simulink model "Guidance_ASMC_T1"  (R2020a)
settings: Solver=ode1  StartTime=0.0  StopTime=120  FixedStep=0.001  RelTol=1e-3
values from neighbouring files (symbols this model uses):
  trayectoria1 = [0 7 15 22 27 30 35 50 57 64 71 78 ... (76 elements, 19x4)]    [Points_T1.mat]
libraries: simulink x5
settings Model: Creator=franc  LastModifiedBy=Sebas
settings SolverCC: ZeroCrossAlgorithm=Adaptive
settings DebuggingCC: IgnoredZcDiagnostic=none
settings ModelReferenceCC: ModelReferenceMinAlgLoopOccurrences=on

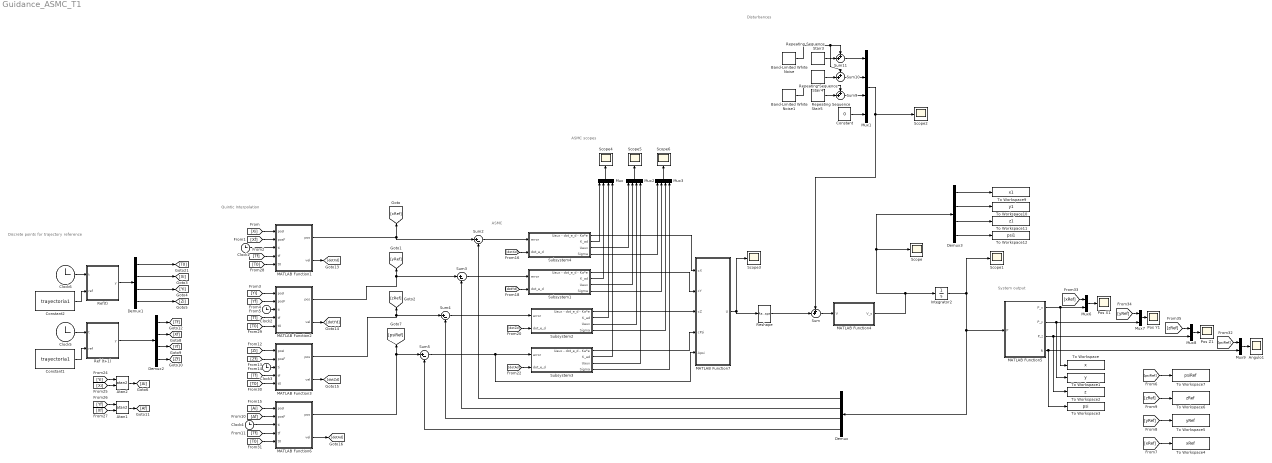
== system Guidance_ASMC_T1 ==
  note: ASMC scopes
  note: Quintic Interpolation
  note: Discrete points for trajectory reference
  note: System output
  note: ASMC
  note: Disturbances
  Angulo1 : Scope
  Atan1 : Trigonometry  Operator=atan2
  Atan2 : Trigonometry  Operator=atan2
  Band-Limited White Noise : simulink/Sources/Band-Limited White Noise  Cov=[1]  Ts=3  seed=[23341]
  Band-Limited White Noise1 : simulink/Sources/Band-Limited White Noise  Cov=[0.5]  Ts=12  seed=[23341]
  Clock{1..6} (6 alike) : Clock
  Constant : Constant  Value=0
  Constant1 : Constant  Value=trayectoria1
  Constant2 : Constant  Value=trayectoria1
  Demux{,1..3} (4 alike) : Demux
  Integrator2 : Integrator
  MATLAB Function1 : MATLAB Function  TreatAsAtomicUnit=on
  MATLAB Function2 : MATLAB Function  TreatAsAtomicUnit=on
  MATLAB Function3 : MATLAB Function  TreatAsAtomicUnit=on
  MATLAB Function4 : MATLAB Function  TreatAsAtomicUnit=on
      settings: MinAlgLoopOccurrences=on
  MATLAB Function5 : MATLAB Function  TreatAsAtomicUnit=on
  MATLAB Function6 : MATLAB Function  TreatAsAtomicUnit=on
  MATLAB Function7 : MATLAB Function  TreatAsAtomicUnit=on
      settings: MinAlgLoopOccurrences=on
  Mux{,1..3} (4 alike) : Mux
  Mux{6..9} (4 alike) : Mux  Inputs=2
  Pos X1 : Scope
  Pos Y1 : Scope
  Pos Z1 : Scope
  Ref (t+1) : MATLAB Function  TreatAsAtomicUnit=on  SystemSampleTime=1
  Ref(t) : MATLAB Function  TreatAsAtomicUnit=on  SystemSampleTime=1
  Repeating Sequence Stair3 : simulink/Sources/Repeating Sequence Stair  OutValues=[1 0.5 -1 -2 -0.5].'  tsamp=24  OutMin=[]  OutMax=[]  OutDataTypeStr=double  OutputDataTypeScalingMode=double  OutDataType=fixdt(0,8)  ConRadixGroup=Best Precision: Vector-wise  OutScaling=2^-12
  Repeating Sequence Stair4 : simulink/Sources/Repeating Sequence Stair  OutValues=[-1 -2 -1.5 -0.5 1].'  tsamp=24  OutMin=[]  OutMax=[]  OutDataTypeStr=double  OutputDataTypeScalingMode=double  OutDataType=fixdt(0,8)  ConRadixGroup=Best Precision: Vector-wise  OutScaling=2^-12
  Repeating Sequence Stair5 : simulink/Sources/Repeating Sequence Stair  OutValues=[0 -0.2 -0.4 -0.6 0].'  tsamp=24  OutMin=[]  OutMax=[]  OutDataTypeStr=double  OutputDataTypeScalingMode=double  OutDataType=fixdt(0,8)  ConRadixGroup=Best Precision: Vector-wise  OutScaling=2^-12
  Reshape : Reshape  OutputDimensionality=Customize  OutputDimensions=[4,1]
  Scope{,1..6} (7 alike) : Scope
  Subsystem1 : Subsystem  mask{Ka=1, K2=1, Beta=1, Mu=0.01}
  Subsystem2 : Subsystem  mask{Ka=2, K2=1, Beta=1, Mu=0.01}
  Subsystem3 : Subsystem  mask{Ka=1, K2=1, Beta=1, Mu=0.01}
  Subsystem4 : Subsystem  mask{Ka=1, K2=1, Beta=1, Mu=0.01}
  Sum{,9..11} (4 alike) : Sum  Inputs=++|
  Sum{2..5} (4 alike) : Sum  Inputs=|+-
  To Workspace : ToWorkspace  VariableName=x  SampleTime=-1
      settings: Save2DSignal=2-D array (concatenate along first dimension)
  To Workspace1 : ToWorkspace  VariableName=y  SampleTime=-1
      settings: Save2DSignal=2-D array (concatenate along first dimension)
  To Workspace10 : ToWorkspace  VariableName=y1  SampleTime=-1
      settings: Save2DSignal=2-D array (concatenate along first dimension)
  To Workspace11 : ToWorkspace  VariableName=z1  SampleTime=-1
      settings: Save2DSignal=2-D array (concatenate along first dimension)
  To Workspace12 : ToWorkspace  VariableName=psi1  SampleTime=-1
      settings: Save2DSignal=2-D array (concatenate along first dimension)
  To Workspace2 : ToWorkspace  VariableName=z  SampleTime=-1
      settings: Save2DSignal=2-D array (concatenate along first dimension)
  To Workspace3 : ToWorkspace  VariableName=psi  SampleTime=-1
      settings: Save2DSignal=2-D array (concatenate along first dimension)
  To Workspace4 : ToWorkspace  VariableName=xRef  SampleTime=-1
      settings: Save2DSignal=2-D array (concatenate along first dimension)
  To Workspace5 : ToWorkspace  VariableName=yRef  SampleTime=-1
      settings: Save2DSignal=2-D array (concatenate along first dimension)
  To Workspace6 : ToWorkspace  VariableName=zRef  SampleTime=-1
      settings: Save2DSignal=2-D array (concatenate along first dimension)
  To Workspace7 : ToWorkspace  VariableName=psiRef  SampleTime=-1
      settings: Save2DSignal=2-D array (concatenate along first dimension)
  To Workspace9 : ToWorkspace  VariableName=x1  SampleTime=-1
      settings: Save2DSignal=2-D array (concatenate along first dimension)
  wires:
  MATLAB Function5/1(P_x) -> Mux6/2, To Workspace/1
  MATLAB Function5/2(P_y) -> Mux7/2, To Workspace1/1
  MATLAB Function5/3(P_z) -> To Workspace2/1, Mux8/2
  MATLAB Function5/4(R) -> Mux9/2, To Workspace3/1
  Mux6/1 -> Pos X1/1
  Mux7/1 -> Pos Y1/1
  Mux8/1 -> Pos Z1/1
  Mux9/1 -> Angulo1/1
  MATLAB Function1/1(pos) -> [xRef], Sum2/1
  MATLAB Function3/1(pos) -> Sum4/1, [zRef]
  MATLAB Function6/1(pos) -> [psiRef], Sum5/1
  MATLAB Function2/1(pos) -> Sum3/1, [yRef]
  [xRef] -> To Workspace4/1
  [yRef] -> To Workspace5/1
  [psiRef] -> To Workspace7/1
  [zRef] -> To Workspace6/1
  [Tf] -> MATLAB Function6/4(tf)
  Clock4/1 -> MATLAB Function6/3(ti)
  [Ai] -> MATLAB Function6/1(posI)
  Demux1/3 -> [Yi]
  [Yf] -> MATLAB Function2/2(posF)
  Clock2/1 -> MATLAB Function2/3(ti)
  [Xi] -> MATLAB Function1/1(posI)
  [Af] -> MATLAB Function6/2(posF)
  [Yi] -> MATLAB Function2/1(posI)
  Demux1/2 -> [Xi]
  Demux2/1 -> [Tf]
  [Tf] -> MATLAB Function2/4(tf)
  Demux1/1 -> [T0]
  [Tf] -> MATLAB Function1/4(tf)
  Demux2/4 -> [Zf]
  Clock1/1 -> MATLAB Function1/3(ti)
  [Tf] -> MATLAB Function3/4(tf)
  [Zf] -> MATLAB Function3/2(posF)
  Clock3/1 -> MATLAB Function3/3(ti)
  [Xf] -> MATLAB Function1/2(posF)
  Demux2/3 -> [Yf]
  [Zi] -> MATLAB Function3/1(posI)
  Demux2/2 -> [Xf]
  MATLAB Function1/2(vel) -> [dotXd]
  MATLAB Function2/2(vel) -> [dotYd]
  MATLAB Function3/2(vel) -> [dotZd]
  MATLAB Function6/2(vel) -> [dotAd]
  Clock5/1 -> Ref (t+1)/1(t)
  Constant1/1 -> Ref (t+1)/2(ref)
  Constant2/1 -> Ref(t)/2(ref)
  Clock6/1 -> Ref(t)/1(t)
  Atan2/1 -> [Ai]
  [Xi] -> Atan2/2
  [Yi] -> Atan2/1
  Atan1/1 -> [Af]
  [Xf] -> Atan1/2
  [Yf] -> Atan1/1
  Ref (t+1)/1(y) -> Demux2/1
  Ref(t)/1(y) -> Demux1/1
  Demux1/4 -> [Zi]
  [T0] -> MATLAB Function1/5(t0)
  [T0] -> MATLAB Function2/5(t0)
  [T0] -> MATLAB Function3/5(t0)
  [T0] -> MATLAB Function6/5(t0)
  [xRef] -> Mux6/1
  [yRef] -> Mux7/1
  [zRef] -> Mux8/1
  [psiRef] -> Mux9/1
  Integrator2/1 -> Scope1/1, Demux/1, MATLAB Function5/1(P)
  Demux/1 -> Sum2/2
  Demux/2 -> Sum3/2
  MATLAB Function7/1(U) -> Reshape/1, Scope3/1
  [dotXd] -> Subsystem4/2(dot_e_d)
  Sum2/1 -> Subsystem4/1(error)
  Sum3/1 -> Subsystem1/1(error)
  Sum4/1 -> Subsystem2/1(error)
  [dotYd] -> Subsystem1/2(dot_e_d)
  [dotZd] -> Subsystem2/2(dot_e_d)
  [dotAd] -> Subsystem3/2(dot_e_d)
  Subsystem4/1(Uaux - dot_e_d - Ka*e) -> MATLAB Function7/1(cX)
  Subsystem1/1(Uaux - dot_e_d - Ka*e) -> MATLAB Function7/2(cY)
  Subsystem2/1(Uaux - dot_e_d - Ka*e) -> MATLAB Function7/3(cZ)
  Subsystem3/1(Uaux - dot_e_d - Ka*e) -> MATLAB Function7/4(cPsi)
  Demux/3 -> Sum4/2
  Demux/4 -> Sum5/2
  Sum5/1 -> Subsystem3/1(error), MATLAB Function7/5(Apsi)
  Sum/1 -> MATLAB Function4/1(V)
  Reshape/1 -> Sum/2
  Sum11/1 -> Mux1/1
  Repeating Sequence Stair4/1 -> Sum10/2
  Sum9/1 -> Mux1/3
  Sum10/1 -> Mux1/2
  Repeating Sequence Stair3/1 -> Sum11/2
  Mux1/1 -> Sum/1, Scope2/1
  Repeating Sequence Stair5/1 -> Sum9/2
  Constant/1 -> Mux1/4
  Band-Limited White Noise/1 -> Sum11/1, Sum10/1
  Band-Limited White Noise1/1 -> Sum9/1
  Demux3/2 -> To Workspace10/1
  Demux3/3 -> To Workspace11/1
  Demux3/4 -> To Workspace12/1
  MATLAB Function4/1(V_s) -> Scope/1, Demux3/1, Integrator2/1
  Demux3/1 -> To Workspace9/1
  Subsystem4/2(K_ad) -> Mux/1
  Subsystem1/2(K_ad) -> Mux/2
  Subsystem2/2(K_ad) -> Mux/3
  Subsystem3/2(K_ad) -> Mux/4
  Subsystem4/3(Uaux) -> Mux2/1
  Subsystem1/3(Uaux) -> Mux2/2
  Subsystem2/3(Uaux) -> Mux2/3
  Subsystem3/3(Uaux) -> Mux2/4
  Subsystem4/4(Sigma) -> Mux3/1
  Subsystem1/4(Sigma) -> Mux3/2
  Subsystem2/4(Sigma) -> Mux3/3
  Subsystem3/4(Sigma) -> Mux3/4
  Mux/1 -> Scope4/1
  Mux2/1 -> Scope5/1
  Mux3/1 -> Scope6/1

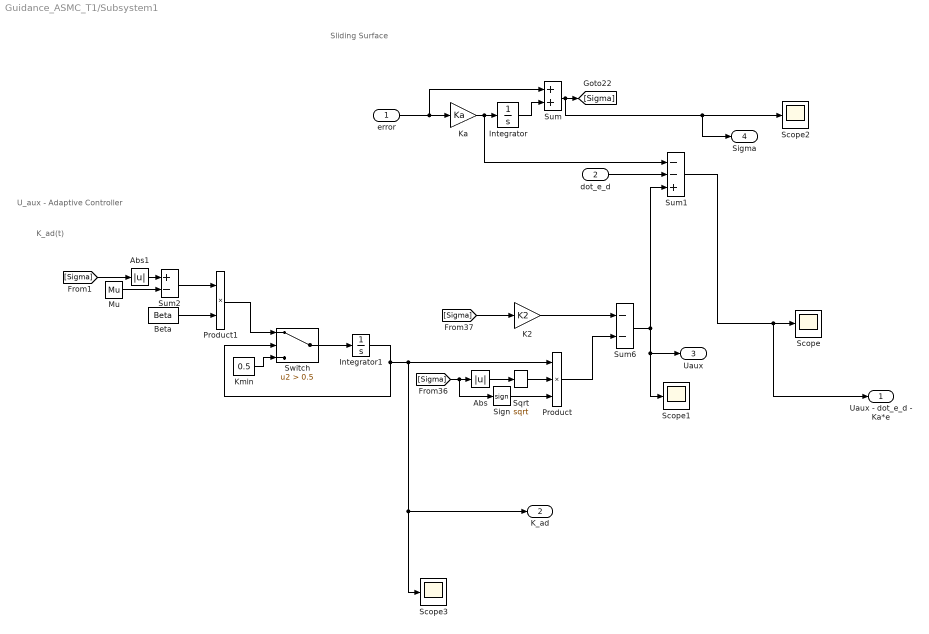
== system Guidance_ASMC_T1/Subsystem1 ==
  note: U_aux - Adaptive Controller
  note: Sliding Surface
  note: K_ad(t)
  error : Inport
  dot_e_d : Inport  Port=2
  Abs : Abs
  Abs1 : Abs
  Beta : Constant  Value=Beta
  Integrator : Integrator
  Integrator1 : Integrator
  K2 : Gain  Gain=K2
  Ka : Gain  Gain=Ka
  Kmin : Constant  Value=0.5
  Mu : Constant  Value=Mu
  Product : Product  Inputs=3
  Product1 : Product
  Scope{,1..3} (4 alike) : Scope
  Sign : Signum
  Sqrt : Sqrt  SaturateOnIntegerOverflow=on
  Sum : Sum
  Sum1 : Sum  Inputs=--+
  Sum2 : Sum  Inputs=+-
  Sum6 : Sum  Inputs=--
  Switch : Switch  Criteria=u2 > Threshold  Threshold=0.5
  Uaux - dot_e_d - Ka*e : Outport
  K_ad : Outport  Port=2
  Uaux : Outport  Port=3
  Sigma : Outport  Port=4
  wires:
  Integrator/1 -> Sum/2
  error/1 -> Sum/1, Ka/1
  [Sigma] -> K2/1
  Ka/1 -> Sum1/1, Integrator/1
  Sum6/1 -> Scope1/1, Uaux/1, Sum1/3
  [Sigma] -> Sign/1, Abs/1
  Product/1 -> Sum6/2
  Abs/1 -> Sqrt/1
  K2/1 -> Sum6/1
  Sum/1 -> Sigma/1, Scope2/1, [Sigma]
  Sign/1 -> Product/3
  Sqrt/1 -> Product/2
  Sum1/1 -> Uaux - dot_e_d - Ka*e/1, Scope/1
  dot_e_d/1 -> Sum1/2
  Switch/1 -> Integrator1/1
  Integrator1/1 -> Scope3/1, K_ad/1, Product/1, Switch/2
  Kmin/1 -> Switch/3
  [Sigma] -> Abs1/1
  Abs1/1 -> Sum2/1
  Mu/1 -> Sum2/2
  Beta/1 -> Product1/2
  Sum2/1 -> Product1/1
  Product1/1 -> Switch/1

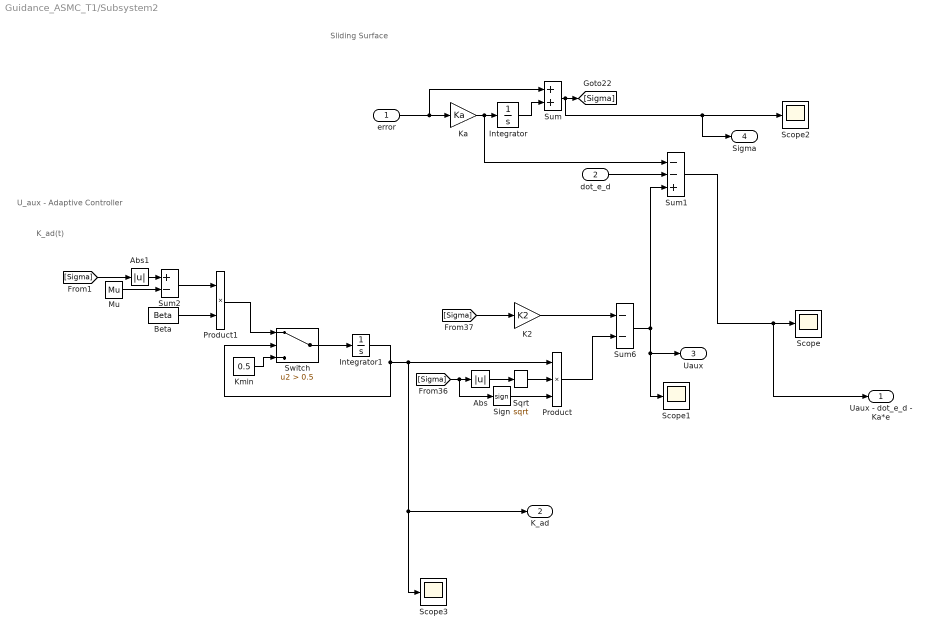
== system Guidance_ASMC_T1/Subsystem2 ==
  note: U_aux - Adaptive Controller
  note: Sliding Surface
  note: K_ad(t)
  error : Inport
  dot_e_d : Inport  Port=2
  Abs : Abs
  Abs1 : Abs
  Beta : Constant  Value=Beta
  Integrator : Integrator
  Integrator1 : Integrator
  K2 : Gain  Gain=K2
  Ka : Gain  Gain=Ka
  Kmin : Constant  Value=0.5
  Mu : Constant  Value=Mu
  Product : Product  Inputs=3
  Product1 : Product
  Scope{,1..3} (4 alike) : Scope
  Sign : Signum
  Sqrt : Sqrt  SaturateOnIntegerOverflow=on
  Sum : Sum
  Sum1 : Sum  Inputs=--+
  Sum2 : Sum  Inputs=+-
  Sum6 : Sum  Inputs=--
  Switch : Switch  Criteria=u2 > Threshold  Threshold=0.5
  Uaux - dot_e_d - Ka*e : Outport
  K_ad : Outport  Port=2
  Uaux : Outport  Port=3
  Sigma : Outport  Port=4
  wires:
  Integrator/1 -> Sum/2
  error/1 -> Sum/1, Ka/1
  [Sigma] -> K2/1
  Ka/1 -> Sum1/1, Integrator/1
  Sum6/1 -> Scope1/1, Uaux/1, Sum1/3
  [Sigma] -> Sign/1, Abs/1
  Product/1 -> Sum6/2
  Abs/1 -> Sqrt/1
  K2/1 -> Sum6/1
  Sum/1 -> Sigma/1, Scope2/1, [Sigma]
  Sign/1 -> Product/3
  Sqrt/1 -> Product/2
  Sum1/1 -> Uaux - dot_e_d - Ka*e/1, Scope/1
  dot_e_d/1 -> Sum1/2
  Switch/1 -> Integrator1/1
  Integrator1/1 -> Scope3/1, K_ad/1, Product/1, Switch/2
  Kmin/1 -> Switch/3
  [Sigma] -> Abs1/1
  Abs1/1 -> Sum2/1
  Mu/1 -> Sum2/2
  Beta/1 -> Product1/2
  Sum2/1 -> Product1/1
  Product1/1 -> Switch/1

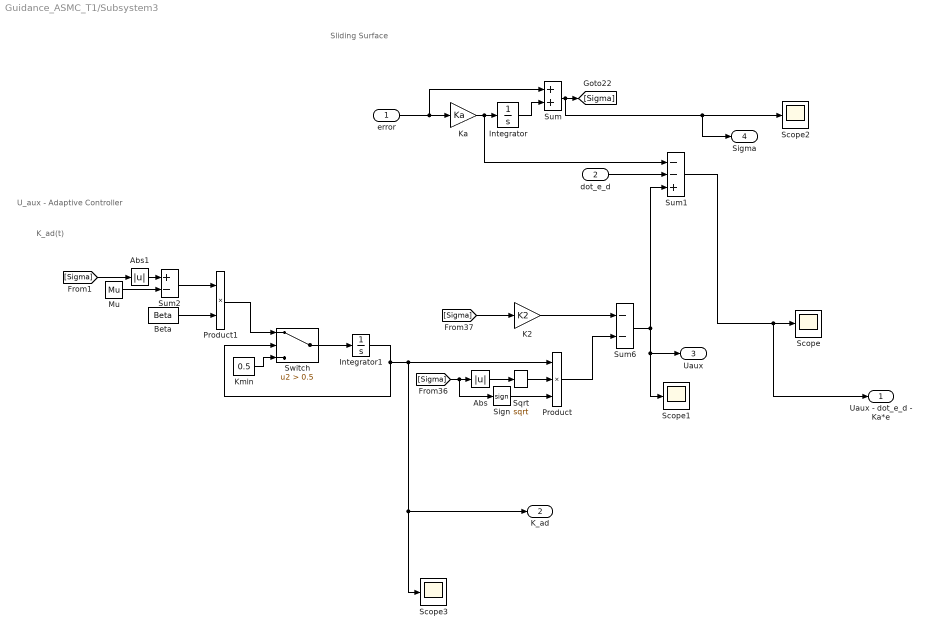
== system Guidance_ASMC_T1/Subsystem3 ==
  note: U_aux - Adaptive Controller
  note: Sliding Surface
  note: K_ad(t)
  error : Inport
  dot_e_d : Inport  Port=2
  Abs : Abs
  Abs1 : Abs
  Beta : Constant  Value=Beta
  Integrator : Integrator
  Integrator1 : Integrator
  K2 : Gain  Gain=K2
  Ka : Gain  Gain=Ka
  Kmin : Constant  Value=0.5
  Mu : Constant  Value=Mu
  Product : Product  Inputs=3
  Product1 : Product
  Scope{,1..3} (4 alike) : Scope
  Sign : Signum
  Sqrt : Sqrt  SaturateOnIntegerOverflow=on
  Sum : Sum
  Sum1 : Sum  Inputs=--+
  Sum2 : Sum  Inputs=+-
  Sum6 : Sum  Inputs=--
  Switch : Switch  Criteria=u2 > Threshold  Threshold=0.5
  Uaux - dot_e_d - Ka*e : Outport
  K_ad : Outport  Port=2
  Uaux : Outport  Port=3
  Sigma : Outport  Port=4
  wires:
  Integrator/1 -> Sum/2
  error/1 -> Sum/1, Ka/1
  [Sigma] -> K2/1
  Ka/1 -> Sum1/1, Integrator/1
  Sum6/1 -> Scope1/1, Uaux/1, Sum1/3
  [Sigma] -> Sign/1, Abs/1
  Product/1 -> Sum6/2
  Abs/1 -> Sqrt/1
  K2/1 -> Sum6/1
  Sum/1 -> Sigma/1, Scope2/1, [Sigma]
  Sign/1 -> Product/3
  Sqrt/1 -> Product/2
  Sum1/1 -> Uaux - dot_e_d - Ka*e/1, Scope/1
  dot_e_d/1 -> Sum1/2
  Switch/1 -> Integrator1/1
  Integrator1/1 -> Scope3/1, K_ad/1, Product/1, Switch/2
  Kmin/1 -> Switch/3
  [Sigma] -> Abs1/1
  Abs1/1 -> Sum2/1
  Mu/1 -> Sum2/2
  Beta/1 -> Product1/2
  Sum2/1 -> Product1/1
  Product1/1 -> Switch/1

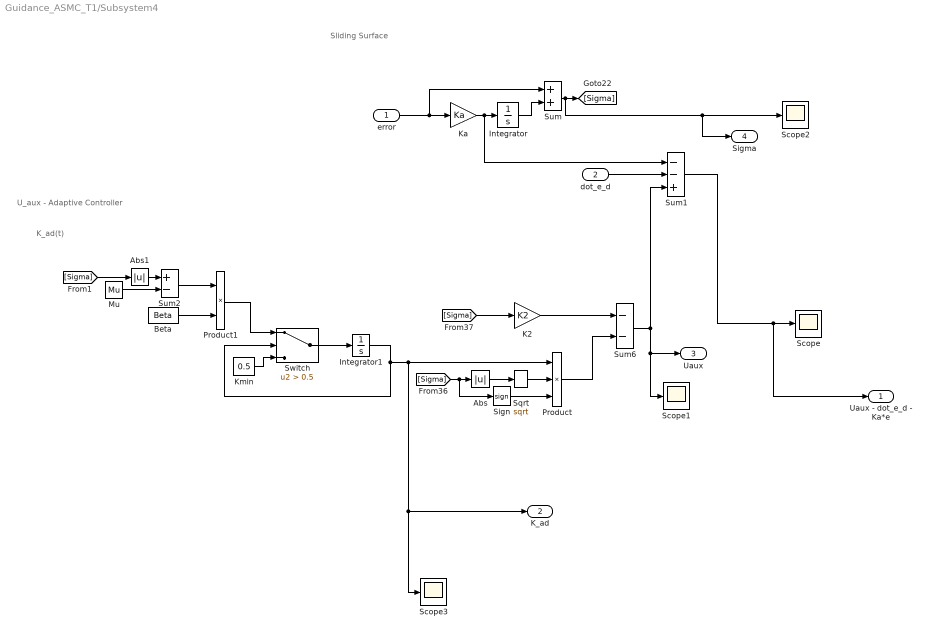
== system Guidance_ASMC_T1/Subsystem4 ==
  note: U_aux - Adaptive Controller
  note: Sliding Surface
  note: K_ad(t)
  error : Inport
  dot_e_d : Inport  Port=2
  Abs : Abs
  Abs1 : Abs
  Beta : Constant  Value=Beta
  Integrator : Integrator
  Integrator1 : Integrator
  K2 : Gain  Gain=K2
  Ka : Gain  Gain=Ka
  Kmin : Constant  Value=0.5
  Mu : Constant  Value=Mu
  Product : Product  Inputs=3
  Product1 : Product
  Scope{,1..3} (4 alike) : Scope
  Sign : Signum
  Sqrt : Sqrt  SaturateOnIntegerOverflow=on
  Sum : Sum
  Sum1 : Sum  Inputs=--+
  Sum2 : Sum  Inputs=+-
  Sum6 : Sum  Inputs=--
  Switch : Switch  Criteria=u2 > Threshold  Threshold=0.5
  Uaux - dot_e_d - Ka*e : Outport
  K_ad : Outport  Port=2
  Uaux : Outport  Port=3
  Sigma : Outport  Port=4
  wires:
  Integrator/1 -> Sum/2
  error/1 -> Sum/1, Ka/1
  [Sigma] -> K2/1
  Ka/1 -> Sum1/1, Integrator/1
  Sum6/1 -> Scope1/1, Uaux/1, Sum1/3
  [Sigma] -> Sign/1, Abs/1
  Product/1 -> Sum6/2
  Abs/1 -> Sqrt/1
  K2/1 -> Sum6/1
  Sum/1 -> Sigma/1, Scope2/1, [Sigma]
  Sign/1 -> Product/3
  Sqrt/1 -> Product/2
  Sum1/1 -> Uaux - dot_e_d - Ka*e/1, Scope/1
  dot_e_d/1 -> Sum1/2
  Switch/1 -> Integrator1/1
  Integrator1/1 -> Scope3/1, K_ad/1, Product/1, Switch/2
  Kmin/1 -> Switch/3
  [Sigma] -> Abs1/1
  Abs1/1 -> Sum2/1
  Mu/1 -> Sum2/2
  Beta/1 -> Product1/2
  Sum2/1 -> Product1/1
  Product1/1 -> Switch/1

== matlab function Guidance_ASMC_T1/MATLAB Function1 ==
  data: posI input; pos output; posF input; ti input; tf input; vel output; t0 input
function [pos,vel] = fcn(posI,posF,ti,tf,t0)

M = [1 t0 t0^2 t0^3 t0^4 t0^5;
    0 1 2*t0 3*t0^2 4*t0^3 5*t0^4;
    0 0 2 6*t0 12*t0^2 20*t0^3;
    1 tf tf^2 tf^3 tf^4 tf^5;
    0 1 2*tf 3*tf^2 4*tf^3 5*tf^4;
    0 0 2 6*tf 12*tf^2 20*tf^3;];
b = [posI;0;0;posF;0;0];
a = M\b;
t = ti;
pos = a(1) + a(2)*t + a(3)*t^2 + a(4)*t^3 + a(5)*t^4 + a(6)*t^5;
vel = a(2) + 2*a(3)*t + 3*a(4)*t^2 + 4*a(5)*t^3 + 5*a(6)*t^4;
end

== matlab function Guidance_ASMC_T1/MATLAB Function2 ==
  data: posI input; pos output; posF input; ti input; tf input; vel output; t0 input
function [pos,vel] = fcn(posI,posF,ti,tf,t0)
%t = tf - t0;
M = [1 t0 t0^2 t0^3 t0^4 t0^5;
    0 1 2*t0 3*t0^2 4*t0^3 5*t0^4;
    0 0 2 6*t0 12*t0^2 20*t0^3;
    1 tf tf^2 tf^3 tf^4 tf^5;
    0 1 2*tf 3*tf^2 4*tf^3 5*tf^4;
    0 0 2 6*tf 12*tf^2 20*tf^3;];
b = [posI;0;0;posF;0;0];
a = M\b;
t = ti;
pos = a(1) + a(2)*t + a(3)*t^2 + a(4)*t^3 + a(5)*t^4 + a(6)*t^5;
vel = a(2) + 2*a(3)*t + 3*a(4)*t^2 + 4*a(5)*t^3 + 5*a(6)*t^4;
end

== matlab function Guidance_ASMC_T1/MATLAB Function3 ==
  data: posI input; pos output; posF input; ti input; tf input; vel output; t0 input
function [pos,vel] = fcn(posI,posF,ti,tf,t0)
%t = tf - t0;
M = [1 t0 t0^2 t0^3 t0^4 t0^5;
    0 1 2*t0 3*t0^2 4*t0^3 5*t0^4;
    0 0 2 6*t0 12*t0^2 20*t0^3;
    1 tf tf^2 tf^3 tf^4 tf^5;
    0 1 2*tf 3*tf^2 4*tf^3 5*tf^4;
    0 0 2 6*tf 12*tf^2 20*tf^3;];
b = [posI;0;0;posF;0;0];
a = M\b;
t = ti;
pos = a(1) + a(2)*t + a(3)*t^2 + a(4)*t^3 + a(5)*t^4 + a(6)*t^5;
vel = a(2) + 2*a(3)*t + 3*a(4)*t^2 + 4*a(5)*t^3 + 5*a(6)*t^4;
end

== matlab function Guidance_ASMC_T1/MATLAB Function6 ==
  data: posI input; pos output; posF input; ti input; tf input; vel output; t0 input
function [pos,vel] = fcn(posI,posF,ti,tf,t0)
%t = tf - t0;
M = [1 t0 t0^2 t0^3 t0^4 t0^5;
    0 1 2*t0 3*t0^2 4*t0^3 5*t0^4;
    0 0 2 6*t0 12*t0^2 20*t0^3;
    1 tf tf^2 tf^3 tf^4 tf^5;
    0 1 2*tf 3*tf^2 4*tf^3 5*tf^4;
    0 0 2 6*tf 12*tf^2 20*tf^3;];
b = [posI;0;0;posF;0;0];
a = M\b;
t = ti;
pos = a(1) + a(2)*t + a(3)*t^2 + a(4)*t^3 + a(5)*t^4 + a(6)*t^5;
vel = a(2) + 2*a(3)*t + 3*a(4)*t^2 + 4*a(5)*t^3 + 5*a(6)*t^4;
end

== matlab function Guidance_ASMC_T1/MATLAB Function4 ==
  data: V input; V_s output
function V_s = Modelo(V)
dotx = V(1,1)*cos(V(4,1)) - V(2,1)*sin(V(4,1));
doty = V(1,1)*sin(V(4,1)) + V(2,1)*cos(V(4,1));
dotz = V(3,1);
W = V(4,1);
V_s = [dotx,doty,dotz,W];

== matlab function Guidance_ASMC_T1/MATLAB Function5 ==
  data: P input; P_x output; P_y output; P_z output; R output
function [P_x,P_y,P_z,R] = Posicion(P)
P_x=P(1,1);
P_y=P(1,2);
P_z=P(1,3);
R=P(1,4);

== matlab function Guidance_ASMC_T1/MATLAB Function7 ==
  data: cX input; U output; cY input; cZ input; cPsi input; Apsi input
function U = G(cX,cY,cZ,cPsi,Apsi)
Aux = [cos(Apsi), sin(Apsi), 0, 0;
       -sin(Apsi), cos(Apsi), 0 , 0;
       0 , 0 , 1 , 0;
       0 , 0 , 0 , 1];
C = [cX,cY,cZ,cPsi]'; 
U = -1*Aux*C;

== matlab function Guidance_ASMC_T1/Ref (t+1) ==
  data: t input; y output; ref input
function y  = fcn(t,ref)
persistent i
if isempty(i)
    i = 2;
end
if t >= ref(i,1)
    i = i + 1;
end
if i < 18
    y = ref(i,:);
else
    y = ref(18,:);
end
end

== matlab function Guidance_ASMC_T1/Ref(t) ==
  data: t input; y output; ref input
function y  = fcn(t,ref)
persistent i
if isempty(i)
    i = 1;
end
if t >= ref(i+1,1)
    i = i + 1;
end
if i < 18
    y = ref(i,:);
else
    y = ref(18,:);
end
end
